simulink library "bpm_dq_S_noH_D_RL_Dyno_16k"  (R2018a)
settings: Solver=VariableStepAuto  StartTime=0.0  StopTime=10.0  RelTol=1e-3
Description:
  | Created by MapleSim.
settings Model: Creator=MapleSim  LastModifiedBy=BEDNASA

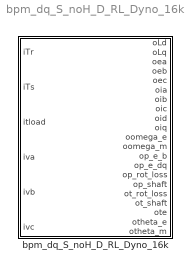
== system bpm_dq_S_noH_D_RL_Dyno_16k ==
  bpm_dq_S_noH_D_RL_Dyno_16k : Subsystem  Description=Subsystem: bpm_dq_S_noH_D_RL_Dyno_16k  mask(bpm_dq_S_noH_D_RL_Dyno_16k){ic=[0., 0., 0., 0.], Par1=.1e-3, Par2=0., Par3=1., Par4=2., Par5=3., Par6=4., Par7=5., Par8=6., Par9=7., Par10=.515e-3, Par11=.884e-1, Par12=.2117e-1, Par13=.2117e-1, Par14=.2117e-1, Par15=.2117e-1, Par16=.2117e-1, Par17=.2117e-1, Par18=.2117e-1, Par19=.2117e-1, Par20=.972e-1, Par21=.2744e-1, Par22=.2777e-1, Par23=.2742e-1, Par24=.2646e-1, Par25=.2426e-1, Par26=.2329e-1, Par27=.2241e-1, Par28=.2241e-1, Par29=3., Par30=0., Par31=1., Par32=12., Par33=19., Par34=26., Par35=35., Par36=41., Par37=56., Par38=0., Par39=.5e3, Par40=.3e4, Par41=.4e4, Par42=.5e4, Par43=.7e4, Par44=.12e5, Par45=.18e5, Par46=1., Par47=.1e2, Par48=9.15, Par49=22., Par50=22., Par51=.2e-3, Par52=.4e-2, Par53=.206e-2, Par54=.1151, ExtData=, MinStep=1/40}
      mask prompts: ic "Initial Conditions:"; Par1 "B:"; Par2 "I_pk0:"; Par3 "I_pk1:"; Par4 "I_pk2:"; Par5 "I_pk3:"; Par6 "I_pk4:"; Par7 "I_pk5:"; Par8 "I_pk6:"; Par9 "I_pk7:"; Par10 "Jrotor:"; Par11 "Ld0:"; Par12 "Ld_a0:"; Par13 "Ld_a1:"; Par14 "Ld_a2:"; Par15 "Ld_a3:"; Par16 "Ld_a4:"; Par17 "Ld_a5:"; Par18 "Ld_a6:"; Par19 "Ld_a7:"; Par20 "Lq0:"; Par21 "Lq_b0:"; Par22 "Lq_b1:"; Par23 "Lq_b2:"; Par24 "Lq_b3:"; Par25 "Lq_b4:"; Par26 "Lq_b5:"; Par27 "Lq_b6:"; Par28 "Lq_b7:"; Par29 "NPP:"; Par30 "Rot_Loss_Power0:"; Par31 "Rot_Loss_Power1:"; Par32 "Rot_Loss_Power2:"; Par33 "Rot_Loss_Power3:"; Par34 "Rot_Loss_Power4:"; Par35 "Rot_Loss_Power5:"; Par36 "Rot_Loss_Power6:"; Par37 "Rot_Loss_Power7:"; Par38 "Rot_Loss_Speed0:"; Par39 "Rot_Loss_Speed1:"; Par40 "Rot_Loss_Speed2:"; Par41 "Rot_Loss_Speed3:"; Par42 "Rot_Loss_Speed4:"; Par43 "Rot_Loss_Speed5:"; Par44 "Rot_Loss_Speed6:"; Par45 "Rot_Loss_Speed7:"; Par46 "Rot_Loss_enable:"; Par47 "Rot_Loss_omega_th:"; Par48 "Rs0:"; Par49 "TrRef:"; Par50 "TsRef:"; Par51 "Ts:"; Par52 "alpha_s:"; Par53 "d_magnet:"; Par54 "phiPM1:"; ExtData "Extended Visualization Data - File Name (leave blank to disable):"; MinStep "Extended Visualization Data - Minimum Sample Step:"
      mask help:
      | Variable Definitions
      |
      | Variable(s) in the Initial Condition Vector:
      |      x[ 0] = `Main.bpm_dq_S_noH_D_RL_Dyno.oid`(t)
      |      x[ 1] = `Main.bpm_dq_S_noH_D_RL_Dyno.oiq`(t)
      |      x[ 2] = `Main.bpm_dq_S_noH_D_RL_Dyno.oomega_e`(t)
      |      x[ 3] = `Main.bpm_dq_S_noH_D_RL_Dyno.otheta_e`(t)
      |
      | Variable(s) in the Output Vector:
      |    oLd:
      |      y[ 0] = `Main.bpm_dq_S_noH_D_RL_Dyno.oLd`(t)
      |    oLq:
      |      y[ 1] = `Main.bpm_dq_S_noH_D_RL_Dyno.oLq`(t)
      |    oea:
      |      y[ 2] = `Main.bpm_dq_S_noH_D_RL_Dyno.oea`(t)
      |    oeb:
      |      y[ 3] = `Main.bpm_dq_S_noH_D_RL_Dyno.oeb`(t)
      |    oec:
      |      y[ 4] = `Main.bpm_dq_S_noH_D_RL_Dyno.oec`(t)
      |    oia:
      |      y[ 5] = `Main.bpm_dq_S_noH_D_RL_Dyno.oia`(t)
      |    oib:
      |      y[ 6] = `Main.bpm_dq_S_noH_D_RL_Dyno.oib`(t)
      |    oic:
      |      y[ 7] = `Main.bpm_dq_S_noH_D_RL_Dyno.oic`(t)
      |    oid:
      |      y[ 8] = `Main.bpm_dq_S_noH_D_RL_Dyno.oid`(t)
      |    oiq:
      |      y[ 9] = `Main.bpm_dq_S_noH_D_RL_Dyno.oiq`(t)
      |    oomega_e:
      |      y[10] = `Main.bpm_dq_S_noH_D_RL_Dyno.oomega_e`(t)
      |    oomega_m:
      |      y[11] = `Main.bpm_dq_S_noH_D_RL_Dyno.oomega_m`(t)
      |    op_e_b:
      |      y[12] = `Main.bpm_dq_S_noH_D_RL_Dyno.op_e_b`(t)
      |    op_e_dq:
      |      y[13] = `Main.bpm_dq_S_noH_D_RL_Dyno.op_e_dq`(t)
      |    op_rot_loss:
      |      y[14] = `Main.bpm_dq_S_noH_D_RL_Dyno.op_rot_loss`(t)
      |    op_shaft:
      |      y[15] = `Main.bpm_dq_S_noH_D_RL_Dyno.op_shaft`(t)
      |    ot_rot_loss:
      |      y[16] = `Main.bpm_dq_S_noH_D_RL_Dyno.ot_rot_loss`(t)
      |    ot_shaft:
      |      y[17] = `Main.bpm_dq_S_noH_D_RL_Dyno.ot_shaft`(t)
      |    ote:
      |      y[18] = `Main.bpm_dq_S_noH_D_RL_Dyno.ote`(t)
      |    otheta_e:
      |      y[19] = `Main.bpm_dq_S_noH_D_RL_Dyno.otheta_e`(t)
      |    otheta_m:
      |      y[20] = `Main.bpm_dq_S_noH_D_RL_Dyno.otheta_m`(t)
      |
      | Variable(s) in the Input Vector:
      |    iTr:
      |      y[ 0] = `Main.bpm_dq_S_noH_D_RL_Dyno.iTr`(t)
      |    iTs:
      |      y[ 1] = `Main.bpm_dq_S_noH_D_RL_Dyno.iTs`(t)
      |    itload:
      |      y[ 2] = `Main.bpm_dq_S_noH_D_RL_Dyno.itload`(t)
      |    iva:
      |      y[ 3] = `Main.bpm_dq_S_noH_D_RL_Dyno.iva`(t)
      |    ivb:
      |      y[ 4] = `Main.bpm_dq_S_noH_D_RL_Dyno.ivb`(t)
      |    ivc:
      |      y[ 5] = `Main.bpm_dq_S_noH_D_RL_Dyno.ivc`(t)
      |
      | Parameter(s):
      |      p[ 0] = `Main.bpm_dq_S_noH_D_RL_Dyno.B` (default = .1e-3)
      |      p[ 1] = `Main.bpm_dq_S_noH_D_RL_Dyno.I_pk0` (default = 0.)
      |      p[ 2] = `Main.bpm_dq_S_noH_D_RL_Dyno.I_pk1` (default = 1.)
      |      p[ 3] = `Main.bpm_dq_S_noH_D_RL_Dyno.I_pk2` (default = 2.)
      |      p[ 4] = `Main.bpm_dq_S_noH_D_RL_Dyno.I_pk3` (default = 3.)
      |      p[ 5] = `Main.bpm_dq_S_noH_D_RL_Dyno.I_pk4` (default = 4.)
      |      p[ 6] = `Main.bpm_dq_S_noH_D_RL_Dyno.I_pk5` (default = 5.)
      |      p[ 7] = `Main.bpm_dq_S_noH_D_RL_Dyno.I_pk6` (default = 6.)
      |      p[ 8] = `Main.bpm_dq_S_noH_D_RL_Dyno.I_pk7` (default = 7.)
      |      p[ 9] = `Main.bpm_dq_S_noH_D_RL_Dyno.Jrotor` (default = .515e-3)
      |      p[10] = `Main.bpm_dq_S_noH_D_RL_Dyno.Ld0` (default = .884e-1)
      |      p[11] = `Main.bpm_dq_S_noH_D_RL_Dyno.Ld_a0` (default = .2117e-1)
      |      p[12] = `Main.bpm_dq_S_noH_D_RL_Dyno.Ld_a1` (default = .2117e-1)
      |      p[13] = `Main.bpm_dq_S_noH_D_RL_Dyno.Ld_a2` (default = .2117e-1)
      |      p[14] = `Main.bpm_dq_S_noH_D_RL_Dyno.Ld_a3` (default = .2117e-1)
      |      p[15] = `Main.bpm_dq_S_noH_D_RL_Dyno.Ld_a4` (default = .2117e-1)
      |      p[16] = `Main.bpm_dq_S_noH_D_RL_Dyno.Ld_a5` (default = .2117e-1)
      |      p[17] = `Main.bpm_dq_S_noH_D_RL_Dyno.Ld_a6` (default = .2117e-1)
      |      p[18] = `Main.bpm_dq_S_noH_D_RL_Dyno.Ld_a7` (default = .2117e-1)
      |      p[19] = `Main.bpm_dq_S_noH_D_RL_Dyno.Lq0` (default = .972e-1)
      |      p[20] = `Main.bpm_dq_S_noH_D_RL_Dyno.Lq_b0` (default = .2744e-1)
      |      p[21] = `Main.bpm_dq_S_noH_D_RL_Dyno.Lq_b1` (default = .2777e-1)
      |      p[22] = `Main.bpm_dq_S_noH_D_RL_Dyno.Lq_b2` (default = .2742e-1)
      |      p[23] = `Main.bpm_dq_S_noH_D_RL_Dyno.Lq_b3` (default = .2646e-1)
      |      p[24] = `Main.bpm_dq_S_noH_D_RL_Dyno.Lq_b4` (default = .2426e-1)
      |      p[25] = `Main.bpm_dq_S_noH_D_RL_Dyno.Lq_b5` (default = .2329e-1)
      |      p[26] = `Main.bpm_dq_S_noH_D_RL_Dyno.Lq_b6` (default = .2241e-1)
      |      p[27] = `Main.bpm_dq_S_noH_D_RL_Dyno.Lq_b7` (default = .2241e-1)
      |      p[28] = `Main.bpm_dq_S_noH_D_RL_Dyno.NPP` (default = 3.)
      |      p[29] = `Main.bpm_dq_S_noH_D_RL_Dyno.Rot_Loss_Power0` (default = 0.)
      |      p[30] = `Main.bpm_dq_S_noH_D_RL_Dyno.Rot_Loss_Power1` (default = 1.)
      |      p[31] = `Main.bpm_dq_S_noH_D_RL_Dyno.Rot_Loss_Power2` (default = 12.)
      |      p[32] = `Main.bpm_dq_S_noH_D_RL_Dyno.Rot_Loss_Power3` (default = 19.)
      |      p[33] = `Main.bpm_dq_S_noH_D_RL_Dyno.Rot_Loss_Power4` (default = 26.)
      |      p[34] = `Main.bpm_dq_S_noH_D_RL_Dyno.Rot_Loss_Power5` (default = 35.)
      |      p[35] = `Main.bpm_dq_S_noH_D_RL_Dyno.Rot_Loss_Power6` (default = 41.)
      |      p[36] = `Main.bpm_dq_S_noH_D_RL_Dyno.Rot_Loss_Power7` (default = 56.)
      |      p[37] = `Main.bpm_dq_S_noH_D_RL_Dyno.Rot_Loss_Speed0` (default = 0.)
      |      p[38] = `Main.bpm_dq_S_noH_D_RL_Dyno.Rot_Loss_Speed1` (default = .5e3)
      |      p[39] = `Main.bpm_dq_S_noH_D_RL_Dyno.Rot_Loss_Speed2` (default = .3e4)
      |      p[40] = `Main.bpm_dq_S_noH_D_RL_Dyno.Rot_Loss_Speed3` (default = .4e4)
      |      p[41] = `Main.bpm_dq_S_noH_D_RL_Dyno.Rot_Loss_Speed4` (default = .5e4)
      |      p[42] = `Main.bpm_dq_S_noH_D_RL_Dyno.Rot_Loss_Speed5` (default = .7e4)
      |      p[43] = `Main.bpm_dq_S_noH_D_RL_Dyno.Rot_Loss_Speed6` (default = .12e5)
      |      p[44] = `Main.bpm_dq_S_noH_D_RL_Dyno.Rot_Loss_Speed7` (default = .18e5)
      |      p[45] = `Main.bpm_dq_S_noH_D_RL_Dyno.Rot_Loss_enable` (default = 1.)
      |      p[46] = `Main.bpm_dq_S_noH_D_RL_Dyno.Rot_Loss_omega_th` (default = .1e2)
      |      p[47] = `Main.bpm_dq_S_noH_D_RL_Dyno.Rs0` (default = 9.15)
      |      p[48] = `Main.bpm_dq_S_noH_D_RL_Dyno.TrRef` (default = 22.)
      |      p[49] = `Main.bpm_dq_S_noH_D_RL_Dyno.TsRef` (default = 22.)
      |      p[50] = `Main.bpm_dq_S_noH_D_RL_Dyno.Ts` (default = .2e-3)
      |      p[51] = `Main.bpm_dq_S_noH_D_RL_Dyno.alpha_s` (default = .4e-2)
      |      p[52] = `Main.bpm_dq_S_noH_D_RL_Dyno.d_magnet` (default = .206e-2)
      |      p[53] = `Main.bpm_dq_S_noH_D_RL_Dyno.phiPM1` (default = .1151)
      mask Help: <!DOCTYPE html PUBLIC "-//W3C//DTD HTML 4.01 Transitional//EN" "http://www.w3.org/TR/1999/REC-html401-19991224/loose.dtd"> <html lang="en"> <head> <title>bpm_dq_S_noH_D_RL_Dyno_16k :: MapleSim model</title> <style type="text/css"> body { background-color: white; margin:10px;} h1 { color: #990000; font-size: x-large; } h2 { color: #990000; font-size: large; margin-top:0ex;     margin-bottom:0ex;   font-weight:bold;  } h3 { color:#990000;  margin-top:0ex;   margin-bottom:0ex;  font-weight:bold;    font-size: medium; } h4 { color:black;    margin-top:0ex;   margin-bottom:0ex;  font-weight:bold;    font-size: medium; } /* Vertical space in tables other than the header and footer banners */ table.body { margin-top: 2ex; margin-bottom: 2ex;} /* Make the text shrink to fit narrow windows, but not stretch too far in wide windows. */ p,h1,h2,div.content div { max-width: 600px; } pre.codeinput { background: #EEEEEE; padding: 10px;} @media print { pre.codeinput { word-wrap:break-word; width:100%; } } span.keyword { color: #0000FF} span.comment { color: #228B22} span.string { color: #A020F0} span.untermstring {color: #B20000} span.syscmd { color: #B28C00} pre.error { color: red;} p.footer { text-align: right; font-size: xx-small; font-weight: lighter; font-style: italic; color: gray; } </style> <meta name="generator" content="DocBook XSL Stylesheets V1.52.2"> <meta name="chunktype" content="refpage"> <meta http-equiv="Content-Script-Type" content="text/javascript"> </head> <body> <a name="top_of_page"></a> <p style="font-size:1px;"> <a name="f8-894621"></a> <a name="transferfcn"></a> <a class="indexterm" name="zmw57dd0e42758"></a></p> <h1 class="reftitle">bpm_dq_S_noH_D_RL_Dyno_16k</h1> <p>Simulink Block generated by MapleSim Connector</p> <p><a name="f8-894627"></a></p> <h1>Description <span class="inlinemediaobject"></span></h1> <p><a class="indexterm" name="zmw57dd0e42781"></a></p> <p>The bpm_dq_S_noH_D_RL_Dyno_16k model runs in the continuous domain and is created in the MapleSim modeling environment. The discrete S-Function block bpm_dq_S_noH_D_RL_Dyno_16k is created using MapleSim Connector. The block is a 6-input, 21-output, 54-parameter system.</p> <p><a name="f8-894641"></a></p> <h1>System Variables</h1> <p>The following variables are used in the S-Function block:</p>  State Variable(s)<dl><dd>x[ 0] = `Main.bpm_dq_S_noH_D_RL_Dyno.oid`(t)</dd></br><dd>x[ 1] = `Main.bpm_dq_S_noH_D_RL_Dyno.oiq`(t)</dd></br><dd>x[ 2] = `Main.bpm_dq_S_noH_D_RL_Dyno.oomega_e`(t)</dd></br><dd>x[ 3] = `Main.bpm_dq_S_noH_D_RL_Dyno.otheta_e`(t)</dd></br></dl> Output Variable(s)<dl><dd>oLd:</dd></br><dd>&nbsp;&nbsp;y[ 0] = `Main.bpm_dq_S_noH_D_RL_Dyno.oLd`(t)</dd></br><dd>oLq:</dd></br><dd>&nbsp;&nbsp;y[ 1] = `Main.bpm_dq_S_noH_D_RL_Dyno.oLq`(t)</dd></br><dd>oea:</dd></br><dd>&nbsp;&nbsp;y[ 2] = `Main.bpm_dq_S_noH_D_RL_Dyno.oea`(t)</dd></br><dd>oeb:</dd></br><dd>&nbsp;&nbsp;y[ 3] = `Main.bpm_dq_S_noH_D_RL_Dyno.oeb`(t)</dd></br><dd>oec:</dd></br><dd>&nbsp;&nbsp;y[ 4] = `Main.bpm_dq_S_noH_D_RL_Dyno.oec`(t)</dd></br><dd>oia:</dd></br><dd>&nbsp;&nbsp;y[ 5] = `Main.bpm_dq_S_noH_D_RL_Dyno.oia`(t)</dd></br><dd>oib:</dd></br><dd>&nbsp;&nbsp;y[ 6] = `Main.bpm_dq_S_noH_D_RL_Dyno.oib`(t)</dd></br><dd>oic:</dd></br><dd>&nbsp;&nbsp;y[ 7] = `Main.bpm_dq_S_noH_D_RL_Dyno.oic`(t)</dd></br><dd>oid:</dd></br><dd>&nbsp;&nbsp;y[ 8] = `Main.bpm_dq_S_noH_D_RL_Dyno.oid`(t)</dd></br><dd>oiq:</dd></br><dd>&nbsp;&nbsp;y[ 9] = `Main.bpm_dq_S_noH_D_RL_Dyno.oiq`(t)</dd></br><dd>oomega_e:</dd></br><dd>&nbsp;&nbsp;y[10] = `Main.bpm_dq_S_noH_D_RL_Dyno.oomega_e`(t)</dd></br><dd>oomega_m:</dd></br><dd>&nbsp;&nbsp;y[11] = `Main.bpm_dq_S_noH_D_RL_Dyno.oomega_m`(t)</dd></br><dd>op_e_b:</dd></br><dd>&nbsp;&nbsp;y[12] = `Main.bpm_dq_S_noH_D_RL_Dyno.op_e_b`(t)</dd></br><dd>op_e_dq:</dd></br><dd>&nbsp;&nbsp;y[13] = `Main.bpm_dq_S_noH_D_RL_Dyno.op_e_dq`(t)</dd></br><dd>op_rot_loss:</dd></br><dd>&nbsp;&nbsp;y[14] = `Main.bpm_dq_S_noH_D_RL_Dyno.op_rot_loss`(t)</dd></br><dd>op_shaft:</dd></br><dd>&nbsp;&nbsp;y[15] = `Main.bpm_dq_S_noH_D_RL_Dyno.op_shaft`(t)</dd></br><dd>ot_rot_loss:</dd></br><dd>&nbsp;&nbsp;y[16] = `Main.bpm_dq_S_noH_D_RL_Dyno.ot_rot_loss`(t)</dd></br><dd>ot_shaft:</dd></br><dd>&nbsp;&nbsp;y[17] = `Main.bpm_dq_S_noH_D_RL_Dyno.ot_shaft`(t)</dd></br><dd>ote:</dd></br><dd>&nbsp;&nbsp;y[18] = `Main.bpm_dq_S_noH_D_RL_Dyno.ote`(t)</dd></br><dd>otheta_e:</dd></br><dd>&nbsp;&nbsp;y[19] = `Main.bpm_dq_S_noH_D_RL_Dyno.otheta_e`(t)</dd></br><dd>otheta_m:</dd></br><dd>&nbsp;&nbsp;y[20] = `Main.bpm_dq_S_noH_D_RL_Dyno.otheta_m`(t)</dd></br></dl> Input Variable(s)<dl><dd>iTr:</dd></br><dd>&nbsp;&nbsp;y[ 0] = `Main.bpm_dq_S_noH_D_RL_Dyno.iTr`(t)</dd></br><dd>iTs:</dd></br><dd>&nbsp;&nbsp;y[ 1] = `Main.bpm_dq_S_noH_D_RL_Dyno.iTs`(t)</dd></br><dd>itload:</dd></br><dd>&nbsp;&nbsp;y[ 2] = `Main.bpm_dq_S_noH_D_RL_Dyno.itload`(t)</dd></br><dd>iva:</dd></br><dd>&nbsp;&nbsp;y[ 3] = `Main.bpm_dq_S_noH_D_RL_Dyno.iva`(t)</dd></br><dd>ivb:</dd></br><dd>&nbsp;&nbsp;y[ 4] = `Main.bpm_dq_S_noH_D_RL_Dyno.ivb`(t)</dd></br><dd>ivc:</dd></br><dd>&nbsp;&nbsp;y[ 5] = `Main.bpm_dq_S_noH_D_RL_Dyno.ivc`(t)</dd></br></dl> Parameter(s)<dl><dd>p[ 0] = `Main.bpm_dq_S_noH_D_RL_Dyno.B` (default = .1e-3)</dd></br><dd>p[ 1] = `Main.bpm_dq_S_noH_D_RL_Dyno.I_pk0` (default = 0.)</dd></br><dd>p[ 2] = `Main.bpm_dq_S_noH_D_RL_Dyno.I_pk1` (default = 1.)</dd></br><dd>p[ 3] = `Main.bpm_dq_S_noH_D_RL_Dyno.I_pk2` (default = 2.)</dd></br><dd>p[ 4] = `Main.bpm_dq_S_noH_D_RL_Dyno.I_pk3` (default = 3.)</dd></br><dd>p[ 5] = `Main.bpm_dq_S_noH_D_RL_Dyno.I_pk4` (default = 4.)</dd></br><dd>p[ 6] = `Main.bpm_dq_S_noH_D_RL_Dyno.I_pk5` (default = 5.)</dd></br><dd>p[ 7] = `Main.bpm_dq_S_noH_D_RL_Dyno.I_pk6` (default = 6.)</dd></br><dd>p[ 8] = `Main.bpm_dq_S_noH_D_RL_Dyno.I_pk7` (default = 7.)</dd></br><dd>p[ 9] = `Main.bpm_dq_S_noH_D_RL_Dyno.Jrotor` (default = .515e-3)</dd></br><dd>p[10] = `Main.bpm_dq_S_noH_D_RL_Dyno.Ld0` (default = .884e-1)</dd></br><dd>p[11] = `Main.bpm_dq_S_noH_D_RL_Dyno.Ld_a0` (default = .2117e-1)</dd></br><dd>p[12] = `Main.bpm_dq_S_noH_D_RL_Dyno.Ld_a1` (default = .2117e-1)</dd></br><dd>p[13] = `Main.bpm_dq_S_noH_D_RL_Dyno.Ld_a2` (default = .2117e-1)</dd></br><dd>p[14] = `Main.bpm_dq_S_noH_D_RL_Dyno.Ld_a3` (default = .2117e-1)</dd></br><dd>p[15] = `Main.bpm_dq_S_noH_D_RL_Dyno.Ld_a4` (default = .2117e-1)</dd></br><dd>p[16] = `Main.bpm_dq_S_noH_D_RL_Dyno.Ld_a5` (default = .2117e-1)</dd></br><dd>p[17] = `Main.bpm_dq_S_noH_D_RL_Dyno.Ld_a6` (default = .2117e-1)</dd></br><dd>p[18] = `Main.bpm_dq_S_noH_D_RL_Dyno.Ld_a7` (default = .2117e-1)</dd></br><dd>p[19] = `Main.bpm_dq_S_noH_D_RL_Dyno.Lq0` (default = .972e-1)</dd></br><dd>p[20] = `Main.bpm_dq_S_noH_D_RL_Dyno.Lq_b0` (default = .2744e-1)</dd></br><dd>p[21] = `Main.bpm_dq_S_noH_D_RL_Dyno.Lq_b1` (default = .2777e-1)</dd></br><dd>p[22] = `Main.bpm_dq_S_noH_D_RL_Dyno.Lq_b2` (default = .2742e-1)</dd></br><dd>p[23] = `Main.bpm_dq_S_noH_D_RL_Dyno.Lq_b3` (default = .2646e-1)</dd></br><dd>p[24] = `Main.bpm_dq_S_noH_D_RL_Dyno.Lq_b4` (default = .2426e-1)</dd></br><dd>p[25] = `Main.bpm_dq_S_noH_D_RL_Dyno.Lq_b5` (default = .2329e-1)</dd></br><dd>p[26] = `Main.bpm_dq_S_noH_D_RL_Dyno.Lq_b6` (default = .2241e-1)</dd></br><dd>p[27] = `Main.bpm_dq_S_noH_D_RL_Dyno.Lq_b7` (default = .2241e-1)</dd></br><dd>p[28] = `Main.bpm_dq_S_noH_D_RL_Dyno.NPP` (default = 3.)</dd></br><dd>p[29] = `Main.bpm_dq_S_noH_D_RL_Dyno.Rot_Loss_Power0` (default = 0.)</dd></br><dd>p[30] = `Main.bpm_dq_S_noH_D_RL_Dyno.Rot_Loss_Power1` (default = 1.)</dd></br><dd>p[31] = `Main.bpm_dq_S_noH_D_RL_Dyno.Rot_Loss_Power2` (default = 12.)</dd></br><dd>p[32] = `Main.bpm_dq_S_noH_D_RL_Dyno.Rot_Loss_Power3` (default = 19.)</dd></br><dd>p[33] = `Main.bpm_dq_S_noH_D_RL_Dyno.Rot_Loss_Power4` (default = 26.)</dd></br><dd>p[34] = `Main.bpm_dq_S_noH_D_RL_Dyno.Rot_Loss_Power5` (default = 35.)</dd></br><dd>p[35] = `Main.bpm_dq_S_noH_D_RL_Dyno.Rot_Loss_Power6` (default = 41.)</dd></br><dd>p[36] = `Main.bpm_dq_S_noH_D_RL_Dyno.Rot_Loss_Power7` (default = 56.)</dd></br><dd>p[37] = `Main.bpm_dq_S_noH_D_RL_Dyno.Rot_Loss_Speed0` (default = 0.)</dd></br><dd>p[38] = `Main.bpm_dq_S_noH_D_RL_Dyno.Rot_Loss_Speed1` (default = .5e3)</dd></br><dd>p[39] = `Main.bpm_dq_S_noH_D_RL_Dyno.Rot_Loss_Speed2` (default = .3e4)</dd></br><dd>p[40] = `Main.bpm_dq_S_noH_D_RL_Dyno.Rot_Loss_Speed3` (default = .4e4)</dd></br><dd>p[41] = `Main.bpm_dq_S_noH_D_RL_Dyno.Rot_Loss_Speed4` (default = .5e4)</dd></br><dd>p[42] = `Main.bpm_dq_S_noH_D_RL_Dyno.Rot_Loss_Speed5` (default = .7e4)</dd></br><dd>p[43] = `Main.bpm_dq_S_noH_D_RL_Dyno.Rot_Loss_Speed6` (default = .12e5)</dd></br><dd>p[44] = `Main.bpm_dq_S_noH_D_RL_Dyno.Rot_Loss_Speed7` (default = .18e5)</dd></br><dd>p[45] = `Main.bpm_dq_S_noH_D_RL_Dyno.Rot_Loss_enable` (default = 1.)</dd></br><dd>p[46] = `Main.bpm_dq_S_noH_D_RL_Dyno.Rot_Loss_omega_th` (default = .1e2)</dd></br><dd>p[47] = `Main.bpm_dq_S_noH_D_RL_Dyno.Rs0` (default = 9.15)</dd></br><dd>p[48] = `Main.bpm_dq_S_noH_D_RL_Dyno.TrRef` (default = 22.)</dd></br><dd>p[49] = `Main.bpm_dq_S_noH_D_RL_Dyno.TsRef` (default = 22.)</dd></br><dd>p[50] = `Main.bpm_dq_S_noH_D_RL_Dyno.Ts` (default = .2e-3)</dd></br><dd>p[51] = `Main.bpm_dq_S_noH_D_RL_Dyno.alpha_s` (default = .4e-2)</dd></br><dd>p[52] = `Main.bpm_dq_S_noH_D_RL_Dyno.d_magnet` (default = .206e-2)</dd></br><dd>p[53] = `Main.bpm_dq_S_noH_D_RL_Dyno.phiPM1` (default = .1151)</dd></br></dl></p> <p><a name="f8-894651"></a></p><h1>Data Type Support</h1> <p>The bpm_dq_S_noH_D_RL_Dyno_16k block accepts inputs and outputs signals of type <tt>double</tt>.</p> <a name="f8-894653"></a><h1>Parameters</h1><dl> <dt><a name="zmw57dd0e42948"></a><b><span class="term">Initial Condition</span>s</b></dt> <dd> <p>The row vector of initial conditions. A vector can be specified to initialize the state variables of the system.</p></dd> <dt><a name="zmw57dd0e42958"></a><span class="term"><b>Parameters</b></span></dt> <dd> <p>The scalars or the row vector of tunable parameters.</p></dd> </dl> <dt><a name="zmw57dd0e42968"></a> </dt><h1>Characteristics</h1> <table cellspacing="0" class="body" cellpadding="4" border="2"><colgroup><col width="41%"><col width="59%"></colgroup><tbody> <tr valign="top"><td bgcolor="#F2F2F2"><p>Direct Feedthrough</p></td><td bgcolor="#F2F2F2"><p>Yes, only if the block has no state variables.</p></td></tr> <tr valign="top"><td bgcolor="#F2F2F2"><p>Sample Time</p></td><td bgcolor="#F2F2F2"><p> Discrete</p></td></tr> <tr valign="top"><td bgcolor="#F2F2F2"><p>Scalar Expansion</p></td><td bgcolor="#F2F2F2"><p>No</p></td></tr> <tr valign="top"><td bgcolor="#F2F2F2"><p>State</p></td><td bgcolor="#F2F2F2"><p>Yes</p></td></tr> <tr valign="top"><td bgcolor="#F2F2F2"><p>Dimensionalized</p></td><td bgcolor="#F2F2F2"><p>Yes</p></td></tr> <tr valign="top"><td bgcolor="#F2F2F2"><p>Zero Crossing</p></td><td bgcolor="#F2F2F2"><p>Yes</p></td></tr> </tbody></table> <p></p><h1>Maple / MapleSim / MapleSim Connector Details</h1> <p></p><dd><p>Maple 2021.1, X86 64 WINDOWS, May 19 2021, Build ID 1539851</p></dd><dd><p>MapleSim 2021.1 Control Design, Wed May 19 23:38:09 EDT 2021, 1539851</p></dd><dd><p>MapleSim 2021.1 Connector for FMI, Wed May 19 23:38:47 EDT 2021, 1539851</p></dd><dd><p>GlobalOptimization 2021.0, Thu Mar 11 13:21:11 EST 2021, 1524228</p></dd><dd><p>MapleSim 2021.1, Wed May 19 23:37:53 EDT 2021, 1539851</p></dd><dd><p>MapleSim 2021.1 Connector, Wed May 19 23:39:01 EDT 2021, 1539851</p></dd><p></p></body></html>
      mask Display: color('blue');text(5,12,'Generated by MapleSim');

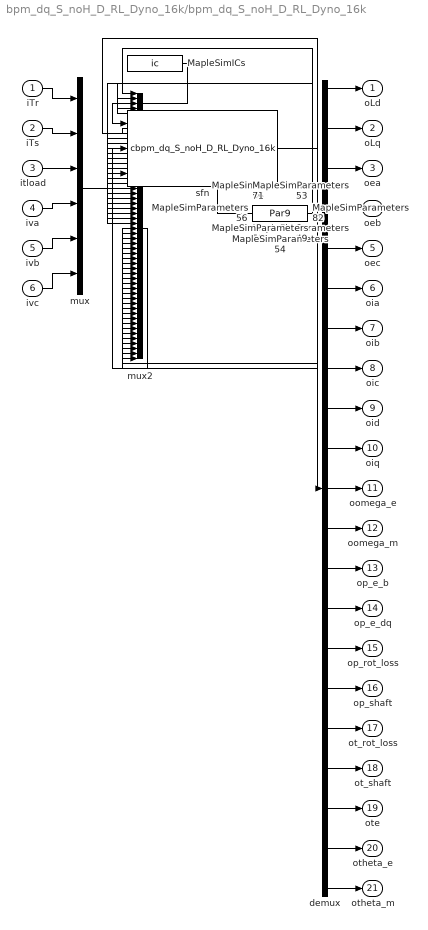
== system bpm_dq_S_noH_D_RL_Dyno_16k/bpm_dq_S_noH_D_RL_Dyno_16k ==
  iTr : Inport
  iTs : Inport  Port=2
  itload : Inport  Port=3
  iva : Inport  Port=4
  ivb : Inport  Port=5
  ivc : Inport  Port=6
  MapleSimICs : Constant  Value=ic
  MapleSimParameters1 : Constant  Value=Par1
  MapleSimParameters10 : Constant  Value=Par10
  MapleSimParameters11 : Constant  Value=Par11
  MapleSimParameters12 : Constant  Value=Par12
  MapleSimParameters13 : Constant  Value=Par13
  MapleSimParameters14 : Constant  Value=Par14
  MapleSimParameters15 : Constant  Value=Par15
  MapleSimParameters16 : Constant  Value=Par16
  MapleSimParameters17 : Constant  Value=Par17
  MapleSimParameters18 : Constant  Value=Par18
  MapleSimParameters19 : Constant  Value=Par19
  MapleSimParameters2 : Constant  Value=Par2
  MapleSimParameters20 : Constant  Value=Par20
  MapleSimParameters21 : Constant  Value=Par21
  MapleSimParameters22 : Constant  Value=Par22
  MapleSimParameters23 : Constant  Value=Par23
  MapleSimParameters24 : Constant  Value=Par24
  MapleSimParameters25 : Constant  Value=Par25
  MapleSimParameters26 : Constant  Value=Par26
  MapleSimParameters27 : Constant  Value=Par27
  MapleSimParameters28 : Constant  Value=Par28
  MapleSimParameters29 : Constant  Value=Par29
  MapleSimParameters3 : Constant  Value=Par3
  MapleSimParameters30 : Constant  Value=Par30
  MapleSimParameters31 : Constant  Value=Par31
  MapleSimParameters32 : Constant  Value=Par32
  MapleSimParameters33 : Constant  Value=Par33
  MapleSimParameters34 : Constant  Value=Par34
  MapleSimParameters35 : Constant  Value=Par35
  MapleSimParameters36 : Constant  Value=Par36
  MapleSimParameters37 : Constant  Value=Par37
  MapleSimParameters38 : Constant  Value=Par38
  MapleSimParameters39 : Constant  Value=Par39
  MapleSimParameters4 : Constant  Value=Par4
  MapleSimParameters40 : Constant  Value=Par40
  MapleSimParameters41 : Constant  Value=Par41
  MapleSimParameters42 : Constant  Value=Par42
  MapleSimParameters43 : Constant  Value=Par43
  MapleSimParameters44 : Constant  Value=Par44
  MapleSimParameters45 : Constant  Value=Par45
  MapleSimParameters46 : Constant  Value=Par46
  MapleSimParameters47 : Constant  Value=Par47
  MapleSimParameters48 : Constant  Value=Par48
  MapleSimParameters49 : Constant  Value=Par49
  MapleSimParameters5 : Constant  Value=Par5
  MapleSimParameters50 : Constant  Value=Par50
  MapleSimParameters51 : Constant  Value=Par51
  MapleSimParameters52 : Constant  Value=Par52
  MapleSimParameters53 : Constant  Value=Par53
  MapleSimParameters54 : Constant  Value=Par54
  MapleSimParameters6 : Constant  Value=Par6
  MapleSimParameters7 : Constant  Value=Par7
  MapleSimParameters8 : Constant  Value=Par8
  MapleSimParameters9 : Constant  Value=Par9
  demux : Demux  Outputs=[1 1 1 1 1 1 1 1 1 1 1 1 1 1 1 1 1 1 1 1 1]
  mux : Mux  Inputs=6
  mux2 : Mux  Inputs=54
  sfn : S-Function  Description=Generated by MapleSim  FunctionName=cbpm_dq_S_noH_D_RL_Dyno_16k  Parameters=ExtData,MinStep  PortCounts=[3, 1]  SFunctionDeploymentMode=off  EnableBusSupport=off
  oLd : Outport
  oLq : Outport  Port=2
  oea : Outport  Port=3
  oeb : Outport  Port=4
  oec : Outport  Port=5
  oia : Outport  Port=6
  oib : Outport  Port=7
  oic : Outport  Port=8
  oid : Outport  Port=9
  oiq : Outport  Port=10
  oomega_e : Outport  Port=11
  oomega_m : Outport  Port=12
  op_e_b : Outport  Port=13
  op_e_dq : Outport  Port=14
  op_rot_loss : Outport  Port=15
  op_shaft : Outport  Port=16
  ot_rot_loss : Outport  Port=17
  ot_shaft : Outport  Port=18
  ote : Outport  Port=19
  otheta_e : Outport  Port=20
  otheta_m : Outport  Port=21
  wires:
  MapleSimICs/1 -> sfn/1
  MapleSimParameters1/1 -> mux2/1
  MapleSimParameters2/1 -> mux2/2
  MapleSimParameters3/1 -> mux2/3
  MapleSimParameters4/1 -> mux2/4
  MapleSimParameters5/1 -> mux2/5
  MapleSimParameters6/1 -> mux2/6
  MapleSimParameters7/1 -> mux2/7
  MapleSimParameters8/1 -> mux2/8
  MapleSimParameters9/1 -> mux2/9
  MapleSimParameters10/1 -> mux2/10
  MapleSimParameters11/1 -> mux2/11
  MapleSimParameters12/1 -> mux2/12
  MapleSimParameters13/1 -> mux2/13
  MapleSimParameters14/1 -> mux2/14
  MapleSimParameters15/1 -> mux2/15
  MapleSimParameters16/1 -> mux2/16
  MapleSimParameters17/1 -> mux2/17
  MapleSimParameters18/1 -> mux2/18
  MapleSimParameters19/1 -> mux2/19
  MapleSimParameters20/1 -> mux2/20
  MapleSimParameters21/1 -> mux2/21
  MapleSimParameters22/1 -> mux2/22
  MapleSimParameters23/1 -> mux2/23
  MapleSimParameters24/1 -> mux2/24
  MapleSimParameters25/1 -> mux2/25
  MapleSimParameters26/1 -> mux2/26
  MapleSimParameters27/1 -> mux2/27
  MapleSimParameters28/1 -> mux2/28
  MapleSimParameters29/1 -> mux2/29
  MapleSimParameters30/1 -> mux2/30
  MapleSimParameters31/1 -> mux2/31
  MapleSimParameters32/1 -> mux2/32
  MapleSimParameters33/1 -> mux2/33
  MapleSimParameters34/1 -> mux2/34
  MapleSimParameters35/1 -> mux2/35
  MapleSimParameters36/1 -> mux2/36
  MapleSimParameters37/1 -> mux2/37
  MapleSimParameters38/1 -> mux2/38
  MapleSimParameters39/1 -> mux2/39
  MapleSimParameters40/1 -> mux2/40
  MapleSimParameters41/1 -> mux2/41
  MapleSimParameters42/1 -> mux2/42
  MapleSimParameters43/1 -> mux2/43
  MapleSimParameters44/1 -> mux2/44
  MapleSimParameters45/1 -> mux2/45
  MapleSimParameters46/1 -> mux2/46
  MapleSimParameters47/1 -> mux2/47
  MapleSimParameters48/1 -> mux2/48
  MapleSimParameters49/1 -> mux2/49
  MapleSimParameters50/1 -> mux2/50
  MapleSimParameters51/1 -> mux2/51
  MapleSimParameters52/1 -> mux2/52
  MapleSimParameters53/1 -> mux2/53
  MapleSimParameters54/1 -> mux2/54
  mux2/1 -> sfn/2
  mux/1 -> sfn/3
  iTr/1 -> mux/1
  iTs/1 -> mux/2
  itload/1 -> mux/3
  iva/1 -> mux/4
  ivb/1 -> mux/5
  ivc/1 -> mux/6
  sfn/1 -> demux/1
  demux/1 -> oLd/1
  demux/2 -> oLq/1
  demux/3 -> oea/1
  demux/4 -> oeb/1
  demux/5 -> oec/1
  demux/6 -> oia/1
  demux/7 -> oib/1
  demux/8 -> oic/1
  demux/9 -> oid/1
  demux/10 -> oiq/1
  demux/11 -> oomega_e/1
  demux/12 -> oomega_m/1
  demux/13 -> op_e_b/1
  demux/14 -> op_e_dq/1
  demux/15 -> op_rot_loss/1
  demux/16 -> op_shaft/1
  demux/17 -> ot_rot_loss/1
  demux/18 -> ot_shaft/1
  demux/19 -> ote/1
  demux/20 -> otheta_e/1
  demux/21 -> otheta_m/1
